simulink model "TestRRT"  (R2018b)
settings: Solver=VariableStepAuto  StartTime=0.0  StopTime=10.0  RelTol=1e-3
undefined symbols (not defined in the file): startPose
libraries: simulink x1
settings Model: Creator=rittwik  LastModifiedBy=rittwik

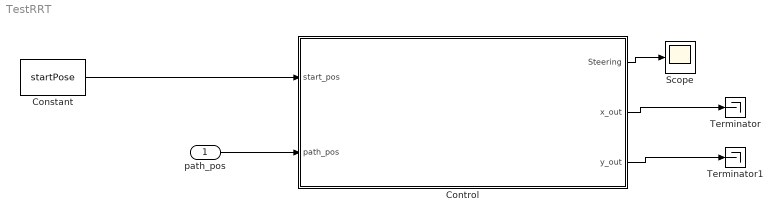
== system TestRRT ==
  path_pos : Inport
  Constant : Constant  Value=startPose
  Control : Subsystem  TreatAsAtomicUnit=on
  Scope : Scope
  Terminator : Terminator
  Terminator1 : Terminator
  wires:
  Control/2(x_out) -> Terminator/1
  Control/3(y_out) -> Terminator1/1
  Control/1(Steering) -> Scope/1
  Constant/1 -> Control/1(start_pos)
  path_pos/1 -> Control/2(path_pos)

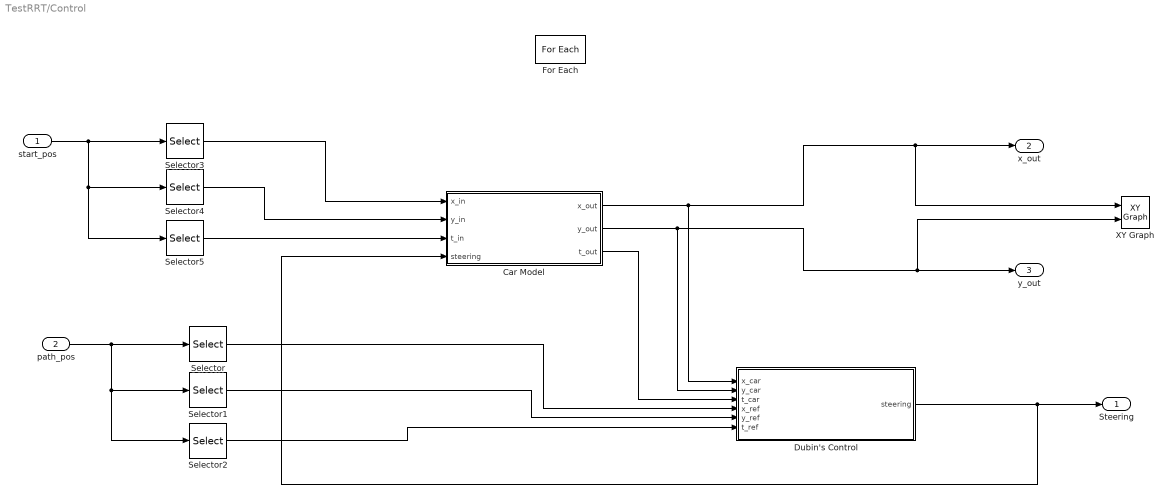
== system TestRRT/Control ==
  start_pos : Inport
  path_pos : Inport  Port=2  Partition=on  PartitionDimension=1  PartitionWidth=1  PartitionOffset=0
  Car Model : Subsystem
  Dubin's Control : Subsystem
  For Each : ForEach  DisableCoverage=on  IndexMode=One-based
  Selector : Selector  InputPortWidth=3  IndexOptions=Index vector (dialog)  Indices=1  OutputSizes=1
  Selector1 : Selector  InputPortWidth=3  IndexOptions=Index vector (dialog)  Indices=2  OutputSizes=1
  Selector2 : Selector  InputPortWidth=3  IndexOptions=Index vector (dialog)  Indices=3  OutputSizes=1
  Selector3 : Selector  InputPortWidth=3  IndexOptions=Index vector (dialog)  Indices=1  OutputSizes=1
  Selector4 : Selector  InputPortWidth=3  IndexOptions=Index vector (dialog)  Indices=2  OutputSizes=1
  Selector5 : Selector  InputPortWidth=3  IndexOptions=Index vector (dialog)  Indices=3  OutputSizes=1
  XY Graph : simulink/Sinks/XY Graph  xmin=-1  xmax=1000  ymin=-1  ymax=1000  st=-1
  Steering : Outport  ConcatenationDimension=1
  x_out : Outport  Port=2  ConcatenationDimension=1
  y_out : Outport  Port=3  ConcatenationDimension=1
  wires:
  Dubin's Control/1(steering) -> Steering/1, Car Model/4(steering)
  Car Model/3(t_out) -> Dubin's Control/3(t_car)
  Selector1/1 -> Dubin's Control/5(y_ref)
  Selector/1 -> Dubin's Control/4(x_ref)
  Car Model/2(y_out) -> Dubin's Control/2(y_car), XY Graph/2, y_out/1
  Car Model/1(x_out) -> Dubin's Control/1(x_car), XY Graph/1, x_out/1
  path_pos/1 -> Selector2/1, Selector1/1, Selector/1
  Selector2/1 -> Dubin's Control/6(t_ref)
  start_pos/1 -> Selector5/1, Selector4/1, Selector3/1
  Selector3/1 -> Car Model/1(x_in)
  Selector4/1 -> Car Model/2(y_in)
  Selector5/1 -> Car Model/3(t_in)

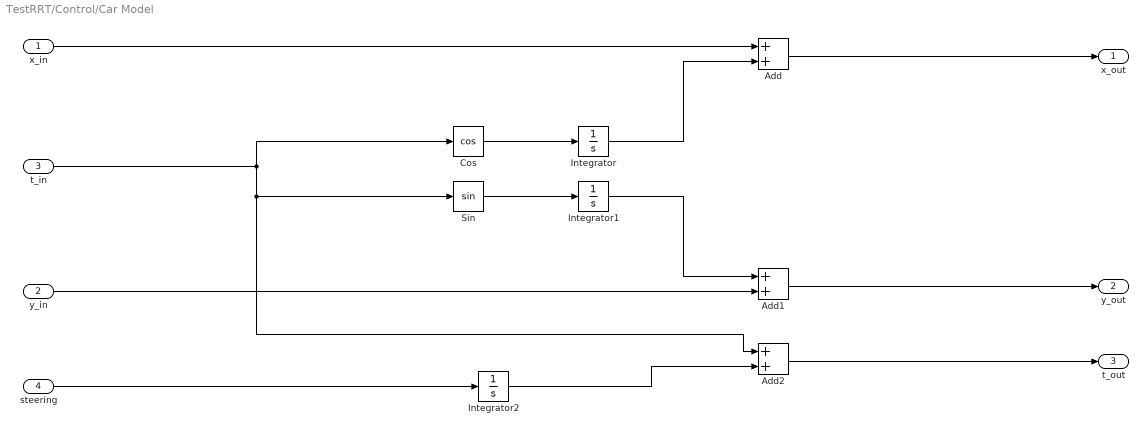
== system TestRRT/Control/Car Model ==
  x_in : Inport
  y_in : Inport  Port=2
  t_in : Inport  Port=3
  steering : Inport  Port=4
  Add : Sum
  Add1 : Sum
  Add2 : Sum
  Cos : Trigonometry  Operator=cos
  Integrator : Integrator
  Integrator1 : Integrator
  Integrator2 : Integrator
  Sin : Trigonometry
  x_out : Outport
  y_out : Outport  Port=2
  t_out : Outport  Port=3
  wires:
  x_in/1 -> Add/1
  Add1/1 -> y_out/1
  Add/1 -> x_out/1
  Integrator/1 -> Add/2
  Cos/1 -> Integrator/1
  t_in/1 -> Cos/1, Add2/1, Sin/1
  Sin/1 -> Integrator1/1
  y_in/1 -> Add1/2
  Integrator1/1 -> Add1/1
  steering/1 -> Integrator2/1
  Integrator2/1 -> Add2/2
  Add2/1 -> t_out/1

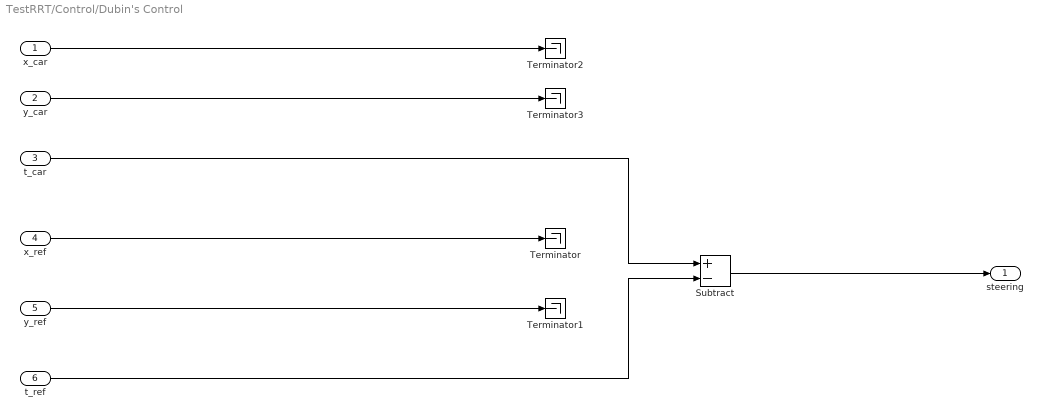
== system TestRRT/Control/Dubin's Control ==
  x_car : Inport
  y_car : Inport  Port=2
  t_car : Inport  Port=3
  x_ref : Inport  Port=4
  y_ref : Inport  Port=5
  t_ref : Inport  Port=6
  Subtract : Sum  Inputs=+-
  Terminator{,1..3} (4 alike) : Terminator
  steering : Outport
  wires:
  t_car/1 -> Subtract/1
  t_ref/1 -> Subtract/2
  Subtract/1 -> steering/1
  y_ref/1 -> Terminator1/1
  x_car/1 -> Terminator2/1
  x_ref/1 -> Terminator/1
  y_car/1 -> Terminator3/1
